simulink model "wireless_charge_model"  (R2024b)
settings: Solver=ode23tb  StartTime=0  StopTime=T_sim  MaxStep=Ts  RelTol=1e-5  AbsTol=1e-7
values from neighbouring files (symbols this model uses):
  f_sw = 85e3    (= 85000)    [wireless_charge_params.m]
  M = k * sqrt(L_p * L_s)    [wireless_charge_params.m]
  R_load = 10    [wireless_charge_params.m]
  V_dc = 100    [wireless_charge_params.m]
settings Model: Creator=DxjCQ  LastModifiedBy=DxjCQ

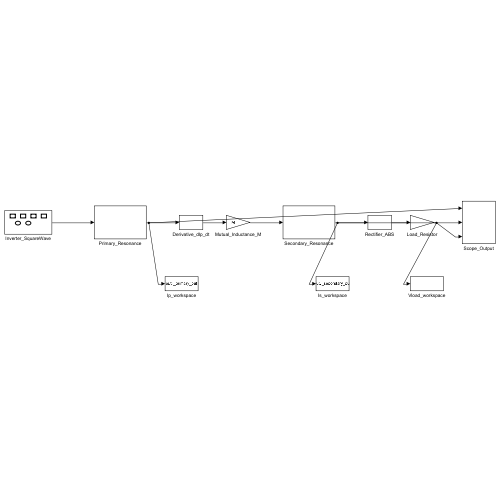
[thumbnail: Simulink's stored preview of the top-level diagram]
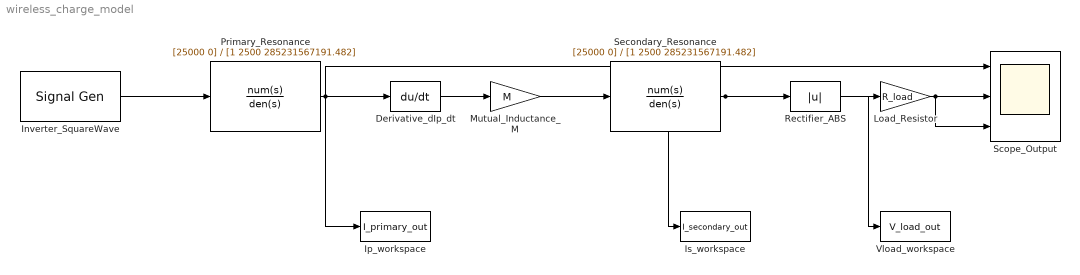
== system wireless_charge_model ==
  Derivative_dIp_dt : Derivative
  Inverter_SquareWave : SignalGenerator  WaveForm=square  Amplitude=V_dc  Frequency=f_sw  Units=rad/sec
  Ip_workspace : ToWorkspace  VariableName=I_primary_out  SampleTime=-1
  Is_workspace : ToWorkspace  VariableName=I_secondary_out  SampleTime=-1
  Load_Resistor : Gain  Gain=R_load
  Mutual_Inductance_M : Gain  Gain=M
  Primary_Resonance : TransferFcn  Numerator=[25000 0]  Denominator=[1 2500 285231567191.482]
  Rectifier_ABS : Abs  SaturateOnIntegerOverflow=off
  Scope_Output : Scope  NumInputPorts=3
  Secondary_Resonance : TransferFcn  Numerator=[25000 0]  Denominator=[1 2500 285231567191.482]
  Vload_workspace : ToWorkspace  VariableName=V_load_out  SampleTime=-1
  wires:
  Inverter_SquareWave/1 -> Primary_Resonance/1
  Primary_Resonance/1 -> Derivative_dIp_dt/1, Scope_Output/1, Ip_workspace/1
  Derivative_dIp_dt/1 -> Mutual_Inductance_M/1
  Mutual_Inductance_M/1 -> Secondary_Resonance/1
  Secondary_Resonance/1 -> Rectifier_ABS/1, Scope_Output/2, Is_workspace/1
  Rectifier_ABS/1 -> Load_Resistor/1
  Load_Resistor/1 -> Scope_Output/3, Vload_workspace/1
